simulink model "Vehicle_model_with_controllers_in_continuous_system_V01"  (R2026a)
settings: Solver=VariableStepAuto  StopTime=inf  RelTol=1e-6
InitFcn:
  | run('Vehicle_parameters_values_V1_MIL.m')
undefined symbols (not defined in the file): Finaldrive, Transmission, Vehicle
libraries: slpidlib x2
(part 2 of 2)

== system Vehicle_model_with_controllers_in_continuous_system_V01/Vehicle_model/Car Plant Model/Vehicle Dynamics/Steering dynamics block ==
  Driver_torque : Inport
  Motor_Voltage : Inport  Port=2
  Add : Sum  Inputs=++-
  EPS_Motor : Subsystem
  Gain : Gain  Gain=1/Vehicle.steering_rack_gear_ratio
  Gain1 : Gain  Gain=180/pi
  Gain2 : Gain  Gain=180/pi
  Gain3 : Gain  Gain=Vehicle.steering_rack_gear_ratio
  K_road : Gain  Gain=3
  Steering Mechanics : Subsystem
  Road_wheel_angle_rad (rad) : Outport
  Road_wheel_angle_deg (theta) : Outport  Port=2
  Steering_wheel_angle_deg (theta) : Outport  Port=3
  tag scope: Assist_motor_torque=global
  wires:
  Add/1 -> Steering Mechanics/1(Total torque)
  Steering Mechanics/1(Steering_wheel_angle_rad (theta)) -> Gain/1, Gain1/1
  K_road/1 -> Add/3, EPS_Motor/2(Road_Torque)  "Road torque"
  Driver_torque/1 -> Add/1  "Driver torque"
  Gain/1 -> K_road/1, Gain2/1, Road_wheel_angle_rad (rad)/1
  EPS_Motor/1(Tm) -> Gain3/1, [Assist_motor_torque]
  Gain1/1 -> Steering_wheel_angle_deg (theta)/1
  Gain2/1 -> Road_wheel_angle_deg (theta)/1
  Motor_Voltage/1 -> EPS_Motor/1(V)  "Motor_voltage"
  Gain3/1 -> Add/2

== system Vehicle_model_with_controllers_in_continuous_system_V01/Vehicle_model/Car Plant Model/Vehicle Dynamics/Total Force block ==
  Wheel torque : Inport
  Brake Pedal : Inport  Port=2
  Grade_angle_deg : Inport  Port=3
  Vehiclespd_m/s : Inport  Port=4
  Add : Sum  Inputs=+--
  Brake Force : Subsystem
  Driving Force : Subsystem
  Resistance Force : Subsystem
  Scope : Scope
      settings: ActiveDisplayYMinimum=434.27496818887704  ActiveDisplayYMaximum=898.01293862748378  DataLoggingVariableName=ScopeData8
  NetForce_N : Outport
  tag scope: Vehicle_Grade_angle=global
  wires:
  Vehiclespd_m/s/1 -> Resistance Force/2(Vehiclespd_m/s)
  Wheel torque/1 -> Driving Force/1(Wheel_torque)
  Brake Force/1(Brake_force) -> Add/2  "BrakeForce_N"
  Driving Force/1(Driving_force) -> Add/1  "DrivingForce_N"
  Grade_angle_deg/1 -> [Vehicle_Grade_angle], Resistance Force/1(Grade_angle_deg)
  Resistance Force/1(Out1) -> Scope/1, Add/3  "ResistanceForce_N"
  Brake Pedal/1 -> Brake Force/1(Brake Pedal)
  Add/1 -> NetForce_N/1  "NetForce_N"

== system Vehicle_model_with_controllers_in_continuous_system_V01/Vehicle_model/Car Plant Model/Vehicle Dynamics/Vehicle Physics ==
  Total_Force : Inport
  Road_wheel_angle : Inport  Port=2
  Force to Speed : Subsystem
  Subsystem : Subsystem
  Vehicle Speed kmph : Outport
  Vehicle_spd_mps : Outport  Port=2
  Yaw_rate_deg/s : Outport  Port=3
  Heading_deg : Outport  Port=4
  x_m : Outport  Port=5
  y_m : Outport  Port=6
  tag scope: Heading_deg=global, Yaw_rate_degps=global, x_posn_m=global, y_posn_m=global
  wires:
  Total_Force/1 -> Force to Speed/1(NetForce_N)  "NetForce_N"
  Force to Speed/1(Vehicle speed_km/hr) -> Vehicle Speed kmph/1
  Force to Speed/2(Vehicle_spd_mps) -> Subsystem/2(Vehicle_spd_mps), Vehicle_spd_mps/1
  Road_wheel_angle/1 -> Subsystem/1(Road_wheel_angle)
  Subsystem/1(Yaw_rate_deg/s) -> [Yaw_rate_degps], Yaw_rate_deg/s/1
  Subsystem/2(Heading_deg) -> [Heading_deg], Heading_deg/1
  Subsystem/3(x) -> [x_posn_m], x_m/1
  Subsystem/4(y) -> [y_posn_m], y_m/1

== system Vehicle_model_with_controllers_in_continuous_system_V01/Vehicle_model/Driver//Controller_I_O/CONTROLLER_I_O/Body ECU ==
  In1 : Inport
  In2 : Inport  Port=2
  Out1 : Outport
  Out2 : Outport  Port=2
  wires:
  In1/1 -> Out1/1
  In2/1 -> Out2/1

== system Vehicle_model_with_controllers_in_continuous_system_V01/Vehicle_model/Driver//Controller_I_O/CONTROLLER_I_O/Implement_ECU ==
  In1 : Inport
  Out1 : Outport
  wires:
  In1/1 -> Out1/1

== system Vehicle_model_with_controllers_in_continuous_system_V01/Vehicle_model/Driver//Controller_I_O/CONTROLLER_I_O/PT_ECU ==
  In1 : Inport
  Out1 : Outport
  wires:
  In1/1 -> Out1/1

== system Vehicle_model_with_controllers_in_continuous_system_V01/Vehicle_model/Driver//Controller_I_O/DRIVER I_O/Drivepdl_interpretor ==
  Driver_pdl : Inport
  Display4 : Display
  Gain : Gain  Gain=-1
  Saturation : Saturate  UpperLimit=100  LowerLimit=0
  Saturation1 : Saturate  UpperLimit=100  LowerLimit=0
  Scope : Scope
      settings: DataLoggingVariableName=ScopeData7
  Drve_Acc_pdl : Outport
  Drvr_Brk_pdl : Outport  Port=2
  tag scope: Driver_pedal_input=global
  wires:
  Driver_pdl/1 -> [Driver_pedal_input], Gain/1, Saturation/1
  Saturation/1 -> Drve_Acc_pdl/1
  Saturation1/1 -> Drvr_Brk_pdl/1
  Gain/1 -> Saturation1/1
  [Driver_pedal_input] -> Display4/1, Scope/1

== system Vehicle_model_with_controllers_in_continuous_system_V01/Vehicle_model/Driver//Controller_I_O/DRIVER I_O/Set_Gear ==
  In1 : Inport
  Display : Display
  Scope : Scope
      settings: DataLoggingVariableName=ScopeData12
  Out1 : Outport
  tag scope: Selected_Gear=global
  wires:
  In1/1 -> [Selected_Gear], Out1/1
  [Selected_Gear] -> Display/1, Scope/1

== system Vehicle_model_with_controllers_in_continuous_system_V01/Vehicle_model/Driver//Controller_I_O/DRIVER I_O/Steering_wheel_angle to Driver_torque ==
  desired angle : Inport
  actual angle : Inport  Port=2  OutDataTypeStr=double
  Display : Display
  Display1 : Display
  Display2 : Display
  Gain : Gain  Gain=0.15
  Scope : Scope
      settings: DataLoggingVariableName=ScopeData6
  Scope1 : Scope
      settings: DataLoggingVariableName=ScopeData10
  Scope2 : Scope
      settings: DataLoggingVariableName=ScopeData11
  Sum : Sum  Inputs=|+-
  Driver_torque : Outport
  tag scope: Actual_steering_wheel_angle=global, Driver_Steering_torque=global, Set_steering_wheel_angle=global
  wires:
  desired angle/1 -> [Set_steering_wheel_angle], Sum/1
  actual angle/1 -> [Actual_steering_wheel_angle], Sum/2
  Sum/1 -> Gain/1
  Gain/1 -> [Driver_Steering_torque], Driver_torque/1
  [Set_steering_wheel_angle] -> Display/1, Scope/1
  [Actual_steering_wheel_angle] -> Display1/1, Scope1/1
  [Driver_Steering_torque] -> Display2/1, Scope2/1

== system Vehicle_model_with_controllers_in_continuous_system_V01/Vehicle_model/Driver//Controller_I_O/DRIVER I_O/Subsystem ==
  In1 : Inport
  In2 : Inport  Port=2
  Out1 : Outport
  Out2 : Outport  Port=2
  wires:
  In1/1 -> Out1/1
  In2/1 -> Out2/1

== system Vehicle_model_with_controllers_in_continuous_system_V01/Vehicle_model/Car Plant Model/Vehicle Dynamics/Steering dynamics block/EPS_Motor ==
  V : Inport
  Road_Torque : Inport  Port=2
  1/Jm : Gain  Gain=1/0.01
  1/L : Gain  Gain=1/0.001
  Add : Sum  Inputs=+--
  Add1 : Sum  Inputs=+--
  Bm : Gain  Gain=0.001
  Gain : Gain  Gain=1/Vehicle.steering_rack_gear_ratio
  Integrator : Integrator
  Integrator1 : Integrator
  Ke : Gain  Gain=0.1
  Kt : Gain  Gain=0.1
  R : Gain  Gain=0.5
  Saturation : Saturate  UpperLimit=2  LowerLimit=-2
  Saturation1 : Saturate  UpperLimit=20  LowerLimit=-20
  Scope : Scope
      settings: ActiveDisplayYMinimum=-0.06671127408147759  ActiveDisplayYMaximum=0.0776635560375095  DataLoggingVariableName=ScopeData13
  Tm : Outport
  wires:
  V/1 -> Add/1  "V"
  Integrator/1 -> Saturation1/1  "current"
  R/1 -> Add/2  "R*i"
  Integrator1/1 -> Ke/1, Bm/1  "speed(w)"
  Ke/1 -> Add/3
  Add/1 -> 1/L/1
  1/L/1 -> Integrator/1
  Kt/1 -> Saturation/1  "Tm"
  Bm/1 -> Add1/2  "Bm*w"
  Add1/1 -> 1/Jm/1
  1/Jm/1 -> Integrator1/1
  Road_Torque/1 -> Gain/1
  Gain/1 -> Scope/1, Add1/3
  Saturation/1 -> Tm/1, Add1/1
  Saturation1/1 -> R/1, Kt/1

== system Vehicle_model_with_controllers_in_continuous_system_V01/Vehicle_model/Car Plant Model/Vehicle Dynamics/Steering dynamics block/Steering Mechanics ==
  Total torque : Inport
  1/J : Gain  Gain=1/0.01
  B : Gain  Gain=0.2
  Integrator : Integrator
  Integrator1 : Integrator
  K : Gain  Gain=5
  Plus : Sum  Inputs=+--
  Steering_wheel_angle_rad (theta) : Outport
  wires:
  1/J/1 -> Integrator/1  "theta_dot_dot"
  Integrator/1 -> B/1, Integrator1/1  "theta_dot"
  Integrator1/1 -> Steering_wheel_angle_rad (theta)/1, K/1  "theta"
  B/1 -> Plus/2  "B*theta_dot"
  K/1 -> Plus/3  "K*theta"
  Plus/1 -> 1/J/1
  Total torque/1 -> Plus/1

== system Vehicle_model_with_controllers_in_continuous_system_V01/Vehicle_model/Car Plant Model/Vehicle Dynamics/Total Force block/Brake Force ==
  note: Output force is proportion of maximum Brake force
      | if input is 0 - no force, 50 - half the max force, 100 - full max force
  Brake Pedal : Inport
  1/100 : Gain  Gain=1/100
  Gain : Gain  Gain=Vehicle.MaxBrakeForce_N
  Brake_force : Outport
  wires:
  Brake Pedal/1 -> 1/100/1
  Gain/1 -> Brake_force/1
  1/100/1 -> Gain/1

== system Vehicle_model_with_controllers_in_continuous_system_V01/Vehicle_model/Car Plant Model/Vehicle Dynamics/Total Force block/Driving Force ==
  Wheel_torque : Inport
  Constant : Constant  Value=Vehicle.wheel_radius
  Divide : Product  Inputs=*/
  Driving_force : Outport
  wires:
  Wheel_torque/1 -> Divide/1
  Divide/1 -> Driving_force/1
  Constant/1 -> Divide/2

== system Vehicle_model_with_controllers_in_continuous_system_V01/Vehicle_model/Car Plant Model/Vehicle Dynamics/Total Force block/Resistance Force ==
  note: Output force is sum of three resistance forces
      | Rolling Resistance
      | Aerodynamic Resistance
      | Grade Resistance
  Grade_angle_deg : Inport
  Vehiclespd_m/s : Inport  Port=2
  Add : Sum  Inputs=+++
  Subsystem : Subsystem
  Subsystem1 : Subsystem
  Subsystem2 : Subsystem
  Out1 : Outport
  wires:
  Add/1 -> Out1/1  "Net_Resistive_Force"
  Vehiclespd_m/s/1 -> Subsystem1/1(Vehiclespd_m/s)
  Subsystem1/1(Aerodrag_resistance_N) -> Add/2  "Aerodrag_resistance_N"
  Subsystem2/1(Grade_resistance_N) -> Add/3  "Grade_resistance_N"
  Grade_angle_deg/1 -> Subsystem2/1(Grade_angle_deg)
  Subsystem/1(Rolling Resistance) -> Add/1  "Rolling_resistance_N"

== system Vehicle_model_with_controllers_in_continuous_system_V01/Vehicle_model/Car Plant Model/Vehicle Dynamics/Vehicle Physics/Force to Speed ==
  NetForce_N : Inport
  Gain1 : Gain  Gain=3.6
  Integrator : Integrator
  Speed_saturation : Saturate  UpperLimit=180  LowerLimit=0
  Vehicle mass : Gain  Gain=1/Vehicle.mass_kg
  Vehicle speed_km/hr : Outport
  Vehicle_spd_mps : Outport  Port=2
  tag scope: Longitudinal_acceleration_mps2=global
  wires:
  Vehicle mass/1 -> [Longitudinal_acceleration_mps2], Integrator/1  "Acceleration"
  NetForce_N/1 -> Vehicle mass/1
  Speed_saturation/1 -> Vehicle_spd_mps/1, Gain1/1
  Integrator/1 -> Speed_saturation/1  "Vehicle speed_m/s"
  Gain1/1 -> Vehicle speed_km/hr/1  "Vehicle speed_km/hr"

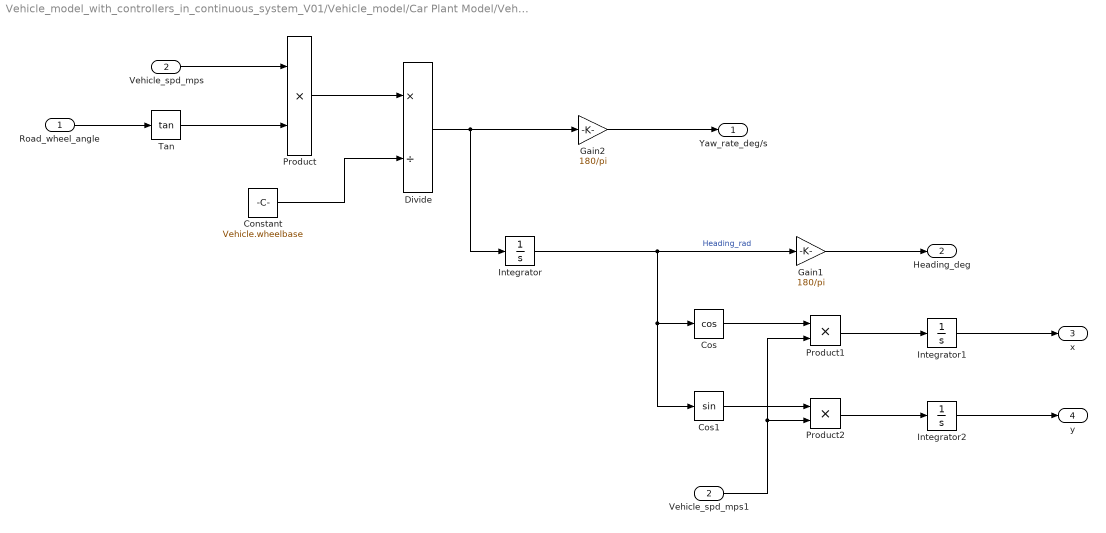
== system Vehicle_model_with_controllers_in_continuous_system_V01/Vehicle_model/Car Plant Model/Vehicle Dynamics/Vehicle Physics/Subsystem ==
  Road_wheel_angle : Inport
  Vehicle_spd_mps : Inport  Port=2
  Constant : Constant  Value=Vehicle.wheelbase
  Cos : Trigonometry  Operator=cos
  Cos1 : Trigonometry
  Divide : Product  Inputs=*/
  Gain1 : Gain  Gain=180/pi
  Gain2 : Gain  Gain=180/pi
  Integrator : Integrator
  Integrator1 : Integrator
  Integrator2 : Integrator
  Product : Product
  Product1 : Product
  Product2 : Product
  Tan : Trigonometry  Operator=tan
  Vehicle_spd_mps1 : InportShadow  Port=2
  Yaw_rate_deg/s : Outport
  Heading_deg : Outport  Port=2
  x : Outport  Port=3
  y : Outport  Port=4
  wires:
  Road_wheel_angle/1 -> Tan/1
  Tan/1 -> Product/2
  Vehicle_spd_mps/1 -> Product/1
  Product/1 -> Divide/1
  Constant/1 -> Divide/2
  Divide/1 -> Integrator/1, Gain2/1
  Integrator/1 -> Cos1/1, Cos/1, Gain1/1  "Heading_rad"
  Cos/1 -> Product1/1
  Vehicle_spd_mps1/1 -> Product2/2, Product1/2
  Cos1/1 -> Product2/1
  Product1/1 -> Integrator1/1
  Product2/1 -> Integrator2/1
  Integrator1/1 -> x/1
  Integrator2/1 -> y/1
  Gain1/1 -> Heading_deg/1
  Gain2/1 -> Yaw_rate_deg/s/1

== system Vehicle_model_with_controllers_in_continuous_system_V01/Vehicle_model/Car Plant Model/Vehicle Dynamics/Total Force block/Resistance Force/Subsystem ==
  Crr : Constant  Value=Vehicle.Crr
  Mass : Constant  Value=Vehicle.mass_kg
  Product : Product  Inputs=3
  g : Constant  Value=Vehicle.g
  Rolling Resistance : Outport
  wires:
  Product/1 -> Rolling Resistance/1
  Mass/1 -> Product/1
  Crr/1 -> Product/2
  g/1 -> Product/3

== system Vehicle_model_with_controllers_in_continuous_system_V01/Vehicle_model/Car Plant Model/Vehicle Dynamics/Total Force block/Resistance Force/Subsystem1 ==
  Vehiclespd_m/s : Inport
  Constant : Constant  Value=0.5
  Constant1 : Constant  Value=Vehicle.rho
  Constant2 : Constant  Value=Vehicle.dragcoeff
  Constant3 : Constant  Value=Vehicle.Area
  Product : Product  Inputs=5
  Square : Math  Operator=square
  Aerodrag_resistance_N : Outport
  wires:
  Vehiclespd_m/s/1 -> Square/1
  Square/1 -> Product/5
  Product/1 -> Aerodrag_resistance_N/1  "Aerodrag_resistance_N"
  Constant/1 -> Product/1
  Constant1/1 -> Product/2
  Constant2/1 -> Product/3
  Constant3/1 -> Product/4

== system Vehicle_model_with_controllers_in_continuous_system_V01/Vehicle_model/Car Plant Model/Vehicle Dynamics/Total Force block/Resistance Force/Subsystem2 ==
  Grade_angle_deg : Inport
  Mass : Constant  Value=Vehicle.mass_kg
  Product : Product  Inputs=3
  Trigonometric Function : Trigonometry
  deg2rad : Gain  Gain=pi/180
  g : Constant  Value=Vehicle.g
  Grade_resistance_N : Outport
  wires:
  deg2rad/1 -> Trigonometric Function/1
  Mass/1 -> Product/1
  Grade_angle_deg/1 -> deg2rad/1
  Product/1 -> Grade_resistance_N/1  "Grade_resistance_N"
  Trigonometric Function/1 -> Product/3
  g/1 -> Product/2

== stateflow chart Vehicle_model_with_controllers_in_continuous_system_V01/Powertrain_ECU/Chart ==
  state READY
    entry:
    Set_spd = Vehicle_spd;
    Cruise_enable=0;
  state OFF
    during:
    Cruise_enable=0;
  state ACTIVE
    during:
    Cruise_enable=1;
  state STANDBY
    during:
    Cruise_enable=0;
  (default) -> OFF
  OFF -> READY : [Cruise_Master_SW==1 && Cr_St==1 && Vehicle_spd>MinCruiseSpd]
  READY -> (junction 19) [order 2]
  READY -> ACTIVE [order 1] : [true]
  (junction 19) -> OFF : [Cruise_Master_SW==0]
  ACTIVE -> (junction 19) [order 2]
  STANDBY -> (junction 19) [order 2]
  ACTIVE -> STANDBY [order 1] : [Cruise_Master_SW==1 && Cr_St==0 || Brk_pdl>0]
  STANDBY -> ACTIVE [order 1] : [Cruise_Master_SW==1 && Cr_St==2]
  data: Cr_St input; Brk_pdl input; Set_spd output; Cruise_enable output; Vehicle_spd input; MinCruiseSpd parameter; Cruise_Master_SW input
